simulink model "modOQPSKconst"  (Simulink 10.1)
settings: Solver=FixedStepDiscrete  StartTime=0.0  StopTime=inf  RelTol=1e-3
libraries: dspsrcs4 x3, commrandsrc3 x2, commfilt2 x2, commutil2 x2, commdigbbndpm3 x1
settings Model: Creator=iba  LastModifiedBy=iba
settings DataIOCC: SaveFormat=Dataset  ReturnWorkspaceOutputs=on
settings OptimizationCC: LifeSpan=auto
settings DebuggingCC: UnderspecifiedInitializationDetection=Simplified  MergeDetectMultiDrivingBlocksExec=error  SFUnexpectedBacktrackingDiag=error  SFNoUnconditionalDefaultTransitionDiag=error  SFExecutionAtInitializationDiag=warning  ArithmeticOperatorsInVariantConditions=error
settings HardwareCC: ProdBitPerPointer=64  ProdBitPerSizeT=64  ProdBitPerPtrDiffT=64  ProdLargestAtomicFloat=Float  ProdIntDivRoundTo=Zero  ProdEndianess=LittleEndian  ProdWordSize=64  ProdHWDeviceType=Intel->x86-64 (Windows64)
settings ModelReferenceCC: PropagateSignalLabelsOutOfModel=on
settings SFSimCC: SimUseLocalCustomCode=on  CustomCodeUndefinedFunction=FilterOut
settings RTWCC: RTWUseLocalCustomCode=on
settings CodeAppCC: StateflowObjectComments=off
settings GRTTargetCC: TargetLangStandard=C99 (ISO)  CombineOutputUpdateFcns=on  GRTInterface=off
settings ConfigComp: CovMetricSettings=dwe  CovHtmlReporting=off  CovSaveCumulativeToWorkspaceVar=off  CovSaveSingleToWorkspaceVar=off  CovExternalEMLEnable=on

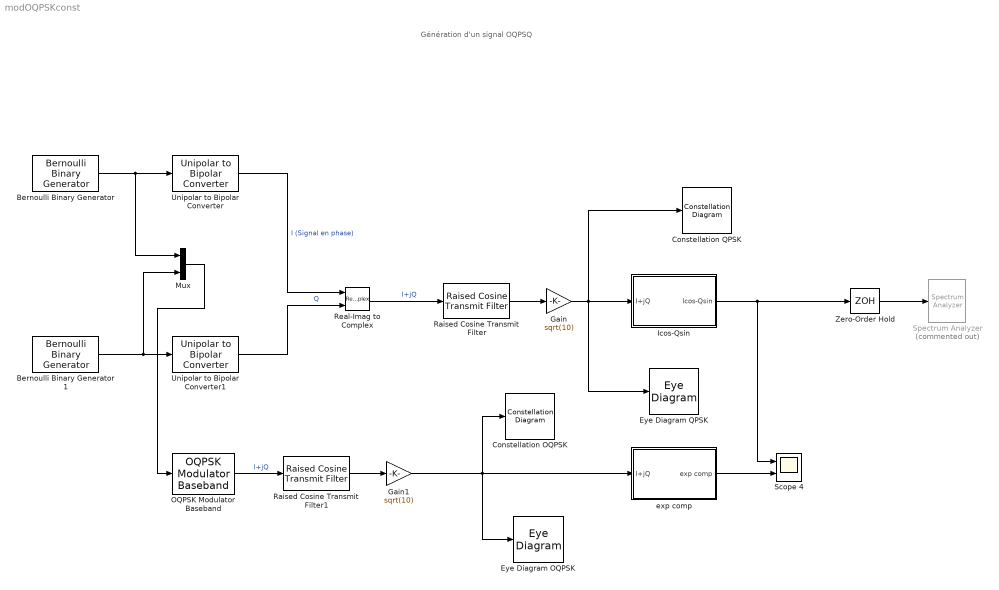
== system modOQPSKconst ==
  note: Génération d'un signal OQPSQ
  "Bernoulli Binary Generator " : commrandsrc3/Bernoulli Binary Generator  ProbabilityOfZero=0.5  SeedSource=Parameter  Seed=62  SampleTime=1  SamplesPerFrame=1  OutputDataType=double  SimulateUsing=Interpreted execution
  Bernoulli Binary Generator 1 : commrandsrc3/Bernoulli Binary Generator  ProbabilityOfZero=0.5  SeedSource=Parameter  Seed=23  SampleTime=1  SamplesPerFrame=1  OutputDataType=double  SimulateUsing=Interpreted execution
  Constellation OQPSK : ConstellationDiagram
  Constellation QPSK : ConstellationDiagram
  Eye Diagram OQPSK : EyeDiagram
  Eye Diagram QPSK : EyeDiagram
  Gain : Gain  Gain=sqrt(10)
  Gain1 : Gain  Gain=sqrt(10)
  Icos-Qsin : Subsystem
  Mux : Mux  Inputs=2
  OQPSK Modulator Baseband : commdigbbndpm3/OQPSK Modulator Baseband  InType=Bit  Ph=0  Mapping=Binary  pulseShape=Half sine  num=[0.7071, 0.7071]  rolloff=0.2  filterSpan=10  sps=2  RateOptions=Allow multirate processing  outDtype=double
      settings: SourceProductBaseCode=CM
  Raised Cosine Transmit Filter : commfilt2/Raised Cosine Transmit Filter  filtType=Square root  R=0.7  filtSpan=10  N=10  filterGain=1  RateOptions=Allow multirate processing  framing=Mute  checkCoeff=off  variableName=rcTxFilt  checkGain=Normalized  sampMode=Mute  saveAsFlag=0  currentFiltSpan=10  D=(10)/2  launchFVT=on  roundingMode=Floor  overflowMode=off  coeffDataTypeStr=Inherit: Same word length as input  coeffMin=[]  coeffMax=[]  coeffLastDataTypeStr=Inherit: Same word length as input  outputDataTypeStr=Inherit: Same as accumulator  outputMin=[]  outputMax=[]  outputLastDataTypeStr=Inherit: Same as accumulator
  Raised Cosine Transmit Filter1 : commfilt2/Raised Cosine Transmit Filter  filtType=Square root  R=0.7  filtSpan=10  N=10  filterGain=1  RateOptions=Allow multirate processing  framing=Mute  checkCoeff=off  variableName=rcTxFilt1  checkGain=Normalized  sampMode=Mute  saveAsFlag=0  currentFiltSpan=10  D=(10)/2  launchFVT=on  roundingMode=Floor  overflowMode=off  coeffDataTypeStr=Inherit: Same word length as input  coeffMin=[]  coeffMax=[]  coeffLastDataTypeStr=Inherit: Same word length as input  outputDataTypeStr=Inherit: Same as accumulator  outputMin=[]  outputMax=[]  outputLastDataTypeStr=Inherit: Same as accumulator
  Real-Imag to Complex : RealImagToComplex
  Scope 4 : Scope  NumInputPorts=2
  Spectrum Analyzer : SpectrumAnalyzer  Commented=on
  Unipolar to Bipolar Converter : commutil2/Unipolar to Bipolar Converter  M=2  polarity=Positive  dataType=Inherit via internal rule
  Unipolar to Bipolar Converter1 : commutil2/Unipolar to Bipolar Converter  M=2  polarity=Positive  dataType=Inherit via internal rule
  Zero-Order Hold : ZeroOrderHold  SampleTime=1/20
  exp comp : Subsystem
  wires:
  Unipolar to Bipolar Converter/1 -> Real-Imag to Complex/1  "I (Signal en phase)"
  "Bernoulli Binary Generator "/1 -> Mux/1, Unipolar to Bipolar Converter/1
  Real-Imag to Complex/1 -> Raised Cosine Transmit Filter/1  "I+jQ"
  Zero-Order Hold/1 -> Spectrum Analyzer/1
  Bernoulli Binary Generator 1/1 -> Mux/2, Unipolar to Bipolar Converter1/1
  Unipolar to Bipolar Converter1/1 -> Real-Imag to Complex/2  "Q"
  Icos-Qsin/1(Icos-Qsin) -> Scope 4/1, Zero-Order Hold/1
  exp comp/1(exp comp) -> Scope 4/2
  Raised Cosine Transmit Filter/1 -> Gain/1
  Gain/1 -> Constellation QPSK/1, Eye Diagram QPSK/1, Icos-Qsin/1(I+jQ)
  Raised Cosine Transmit Filter1/1 -> Gain1/1
  OQPSK Modulator Baseband/1 -> Raised Cosine Transmit Filter1/1  "I+jQ"
  Gain1/1 -> Eye Diagram OQPSK/1, Constellation OQPSK/1, exp comp/1(I+jQ)
  Mux/1 -> OQPSK Modulator Baseband/1

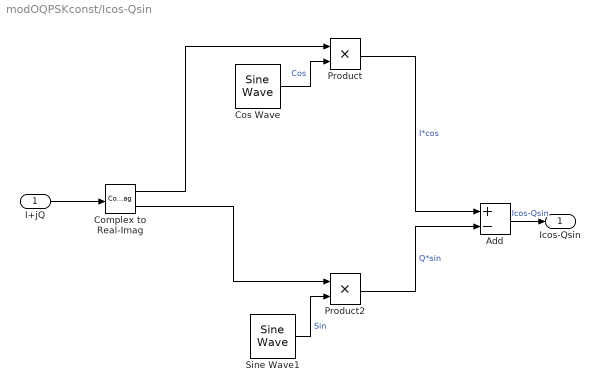
== system modOQPSKconst/Icos-Qsin ==
  I+jQ : Inport
  Add : Sum  Inputs=+-
  Complex to Real-Imag : ComplexToRealImag
  Cos Wave : dspsrcs4/Sine Wave  Amplitude=1  Frequency=5  Phase=pi/2  SampleMode=Discrete  OutComplex=Real  CompMethod=Trigonometric fcn  TableSize=Speed  SampleTime=1/100  SamplesPerFrame=1  ResetState=Restart at time zero  OutputFrames=off  dataType=double  wordLen=16  udDataType=sfix(16)  fracBitsMode=Best precision  numFracBits=15  OutDataTypeStr=double  LastOutDataTypeStr=double
  Product : Product
  Product2 : Product
  Sine Wave1 : dspsrcs4/Sine Wave  Amplitude=1  Frequency=5  Phase=0  SampleMode=Discrete  OutComplex=Real  CompMethod=Trigonometric fcn  TableSize=Speed  SampleTime=1/100  SamplesPerFrame=1  ResetState=Restart at time zero  OutputFrames=off  dataType=double  wordLen=16  udDataType=sfix(16)  fracBitsMode=Best precision  numFracBits=15  OutDataTypeStr=double  LastOutDataTypeStr=double
  Icos-Qsin : Outport
  wires:
  I+jQ/1 -> Complex to Real-Imag/1
  Sine Wave1/1 -> Product2/2  "Sin"
  Product2/1 -> Add/2  "Q*sin"
  Cos Wave/1 -> Product/2  "Cos"
  Complex to Real-Imag/2 -> Product2/1
  Product/1 -> Add/1  "I*cos"
  Complex to Real-Imag/1 -> Product/1
  Add/1 -> Icos-Qsin/1  "Icos-Qsin"

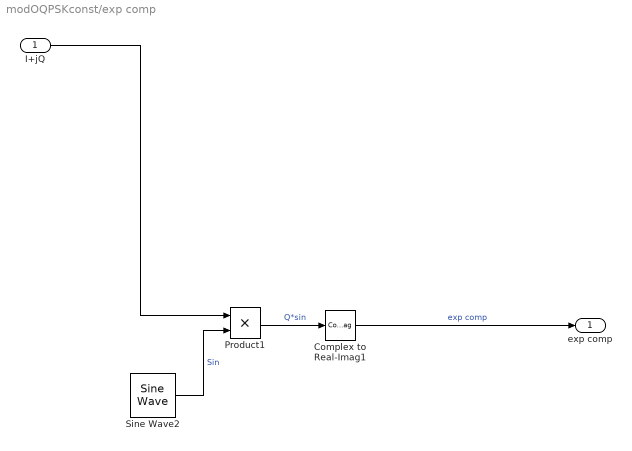
== system modOQPSKconst/exp comp ==
  I+jQ : Inport
  Complex to Real-Imag1 : ComplexToRealImag  Output=Real
  Product1 : Product
  Sine Wave2 : dspsrcs4/Sine Wave  Amplitude=1  Frequency=5  Phase=0  SampleMode=Discrete  OutComplex=Complex  CompMethod=Trigonometric fcn  TableSize=Speed  SampleTime=1/100  SamplesPerFrame=1  ResetState=Restart at time zero  OutputFrames=off  dataType=double  wordLen=16  udDataType=sfix(16)  fracBitsMode=Best precision  numFracBits=15  OutDataTypeStr=double  LastOutDataTypeStr=double
  exp comp : Outport
  wires:
  Sine Wave2/1 -> Product1/2  "Sin"
  Complex to Real-Imag1/1 -> exp comp/1  "exp comp"
  Product1/1 -> Complex to Real-Imag1/1  "Q*sin"
  I+jQ/1 -> Product1/1
